simulink model "tesina"  (R2024b)
settings: Solver=VariableStepAuto  StartTime=0.0  StopTime=3  RelTol=1e-3
undefined symbols (not defined in the file or in its folder): ci_core, ci_energia, ci_omp, ci_T_core, ci_T_omp, ci_T_tar, ci_tar, ion, k0, Lz_valuesAzoto, P_tot
libraries: slpidlib x3, simulink x1
settings Model: Creator=feder  LastModifiedBy=costa

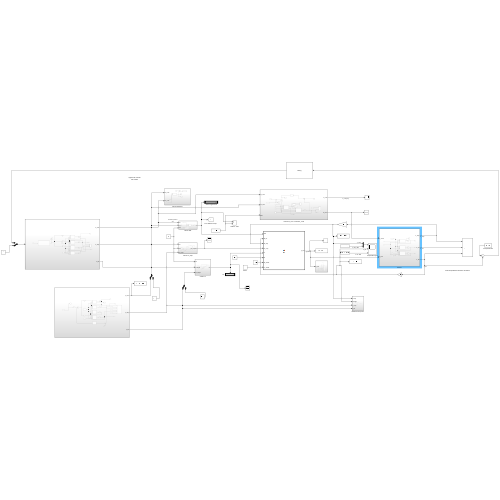
[thumbnail: Simulink's stored preview of the top-level diagram]
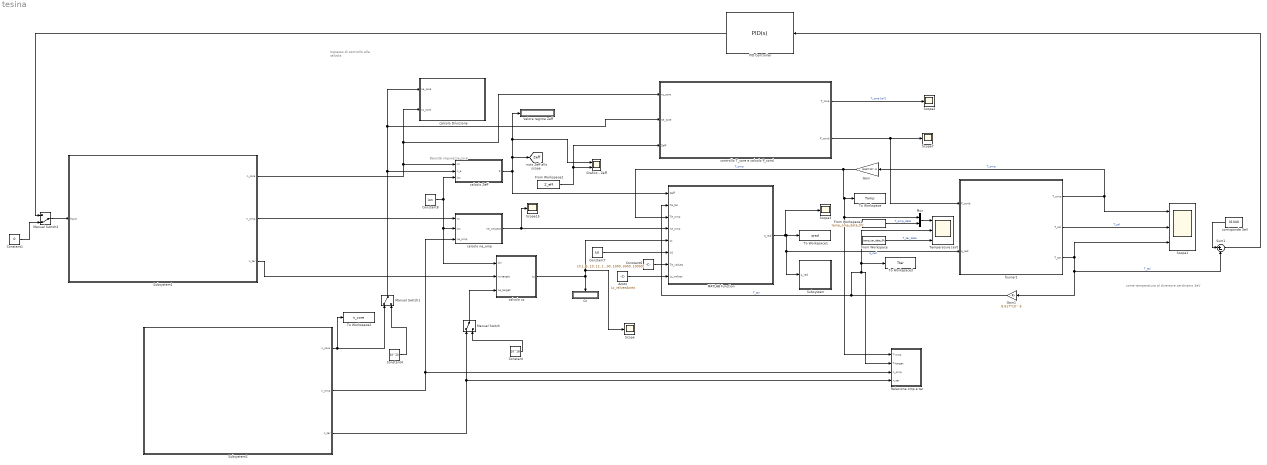
== system tesina ==
  note: come temperatura al divertore cerchiamo 3eV
  note: Ingresso di controllo
      | alla valvola
  note: Densità impurezze
      | core
  Azoto : Constant  Value=Lz_valuesAzoto
  Constant : Constant  Value=10^18
  Constant1 : Constant  Value=0
  Constant4 : Constant  Value=10^20
  Constant6 : Constant  Value=[0,1, 5, 10, 12, 15, 20, 30, 59, 100, 155, 200, 300, 500, 700, 1000, 3000, 10000]
  Constant7 : Constant  Value=k0
  Constant8 : Constant  Value=ion
  Cz : Display
  From Workspace : FromWorkspace  VariableName=temp_tar_data_filt
  From Workspace1 : FromWorkspace  VariableName=temp_omp_data_filt
  From Workspace2 : FromWorkspace  VariableName=Z_eff
  Gain : Gain  Gain=8.617*10^-5
  Gain1 : Gain  Gain=8.617*10^-5
  Grafico - Zeff : Scope  NumInputPorts=2
  MATLAB Function : MATLAB Function  TreatAsAtomicUnit=on
  Manual Switch : ManualSwitch
  Manual Switch1 : ManualSwitch
  Manual Switch2 : ManualSwitch  CurrentSetting=0
  Mux : Mux  Inputs=2
  PID Controller : slpidlib/PID Controller  Controller=PID  Form=Parallel  TimeDomain=Continuous-time  UseExternalTs=off  SampleTime=-1  IntegratorMethod=Forward Euler  FilterMethod=Forward Euler  ControllerParametersSource=internal  P=-5*10^10  I=-0.5*10^8  UseKiTs=off  D=-10^11  UseExternalDerivativeSource=off  N=100  UseFilter=on  TunerSelectOption=Transfer Function Based (PID Tuner App)  InitialConditionSource=internal  InitialConditionForIntegrator=0  InitialConditionForFilter=0  DifferentiatorICPrevScaledInput=0  ExternalReset=none  TrackingMode=off  Kt=1  LimitOutput=off  SatLimitsSource=internal  UpperSaturationLimit=inf  LowerSaturationLimit=-inf  LinearizeAsGain=on  AntiWindupMode=none  Kb=1  LimitIntegrator=off  UpperIntegratorSaturationLimit=inf  LowerIntegratorSaturationLimit=-inf  POutMin=[]  POutMax=[]  IOutMin=[]  IOutMax=[]  DOutMin=[]  DOutMax=[]  NOutMin=[]  NOutMax=[]  SumOutMin=[]  SumOutMax=[]  SaturationOutMin=[]  SaturationOutMax=[]  PParamMin=[]  PParamMax=[]  IParamMin=[]  IParamMax=[]  DParamMin=[]  DParamMax=[]  NParamMin=[]  NParamMax=[]  KbParamMin=[]  KbParamMax=[]  KtParamMin=[]  KtParamMax=[]  KbOutMin=[]  KbOutMax=[]  KtOutMin=[]  KtOutMax=[]  IntegratorOutMin=[]  IntegratorOutMax=[]  FilterOutMin=[]  FilterOutMax=[]  SumI1OutMin=[]  SumI1OutMax=[]  SumI2OutMin=[]  SumI2OutMax=[]  SumI3OutMin=[]  SumI3OutMax=[]  SumI4OutMin=[]  SumI4OutMax=[]  SumDOutMin=[]  SumDOutMax=[]  DifferentiatorOutMin=[]  DifferentiatorOutMax=[]  FilterDiffOutCoefMin=[]  FilterDiffOutCoefMax=[]  ReciprocalOutMin=[]  ReciprocalOutMax=[]  SumDenOutMin=[]  SumDenOutMax=[]  SumNumOutMin=[]  SumNumOutMax=[]  DivideOutMin=[]  DivideOutMax=[]  UdiffTsProdOutMin=[]  UdiffTsProdOutMax=[]  NTsProdOutMin=[]  NTsProdOutMax=[]  UintegralTsProdOutMin=[]  UintegralTsProdOutMax=[]  UngainTsProdOutMin=[]  UngainTsProdOutMax=[]  ClampingZeroOutDataTypeStr=Inherit: Inherit via back propagation  ClampingZeroOutMin=[]  ClampingZeroOutMax=[]  FilterDenConstantOutDataTypeStr=Inherit: Inherit via back propagation  FilterDenConstantOutMin=[]  FilterDenConstantOutMax=[]  PCopyOutDataTypeStr=Inherit: Inherit via back propagation  PCopyOutMin=[]  PCopyOutMax=[]  NCopyOutDataTypeStr=Inherit: Inherit via back propagation  NCopyOutMin=[]  NCopyOutMax=[]  IntegratorContinuousStateAttributes=''  IntegratorStateMustResolveToSignalObject=off  IntegratorRTWStateStorageClass=Auto  FilterContinuousStateAttributes=''  FilterStateMustResolveToSignalObject=off  FilterRTWStateStorageClass=Auto  ParallelPVariant=InternalParameters  IdealPVariant=Disabled  IVariant=InternalParameters  DVariant=InternalParameters  IntegratorVariant=Continuous  SatVariant=Disabled  AWVariant=Passthrough  PCopyVariant=Disabled  TRVariant=Disabled  FdbkBlocksVariant=Forward  IdealPFdbkVariant=Disabled  SatFdbkVariant=Disabled  DerivativeFilterVariant=ContFilter  NVariant=InternalParameters  NCopyVariant=Disabled  FilterICVariant=InternalICsFilter  IntegratorICVariant=InternalICs  ExternalResetVariant=Disabled  TRSumVariant=Passthrough  SumFdbkVariant=Disabled  SumVariant=Sum_PID  TsampFilterVariant=InternalTs  TsampNgainVariant=Passthrough  TsampIntegralVariant=Disabled_SignalSpec  ExternalSaturationOutDataTypeStr=Inherit: Same as second input  DerivativeSourceVariant=ErrorSignal  PreIntVariant=InternalPreInt
  Relazione omp e tar : Subsystem
  Scope{,2..3,7,15} (5 alike) : Scope
  Scope1 : Scope  NumInputPorts=3
  Subsystem : Subsystem
  Subsystem1 : Subsystem
  Subsystem2 : Subsystem
  Sum1 : Sum  Inputs=|+-
  Temperature [eV] : Scope  NumInputPorts=3
  To Workspace : ToWorkspace  VariableName=Tomp  SaveFormat=Timeseries  SampleTime=-1
  To Workspace1 : ToWorkspace  VariableName=qrad  SaveFormat=Timeseries  SampleTime=-1
  To Workspace2 : ToWorkspace  VariableName=n_core  SaveFormat=Timeseries  SampleTime=-1
  To Workspace3 : ToWorkspace  VariableName=Ttar  SaveFormat=Timeseries  SampleTime=-1
  Valore regime Zeff : Display
  calcolo Diluizione : Subsystem
  calcolo Zeff : Subsystem
  calcolo cz : Subsystem
  calcolo ne_omp : Subsystem
  controllo T_core e calcolo P_cond : Subsystem
  corrisponde 3eV : Constant  Value=31340
  fourier1 : Subsystem
  tag scope: Zeff=global
  wires:
  Gain/1 -> MATLAB Function/3(Te_omp), Mux/1, Relazione omp e tar/1(T-omp), To Workspace/1  "T_omp"
  PID Controller/1 -> Manual Switch2/1
  From Workspace1/1 -> Mux/2  "T_omp_data"
  Subsystem2/2(n_omp) -> calcolo ne_omp/3(ne_omp), Relazione omp e tar/3(n_omp)
  Subsystem1/2(n_omp) -> calcolo ne_omp/1(nz)
  Gain1/1 -> Relazione omp e tar/2(T-target), Temperature [eV]/2, To Workspace3/1, MATLAB Function/2(Te_tar)  "T_tar"
  Azoto/1 -> MATLAB Function/8(Lz_values)
  controllo T_core e calcolo P_cond/2(P_cond) -> fourier1/1(P_cond), Scope7/1
  Manual Switch2/1 -> Subsystem1/1(Input)
  Manual Switch/1 -> calcolo cz/3(ne_target)
  Subsystem1/3(n_tar) -> calcolo cz/2(nz-target)
  Subsystem2/3(n_tar) -> Manual Switch/1, Relazione omp e tar/4(n_tar)
  From Workspace2/1 -> controllo T_core e calcolo P_cond/3(Zeff), Grafico - Zeff/2
  Manual Switch1/1 -> controllo T_core e calcolo P_cond/2(ne_core), calcolo Diluizione/1(ne_core), calcolo Zeff/2(n_e)
  Subsystem2/1(n_core) -> Manual Switch1/1, To Workspace2/1
  controllo T_core e calcolo P_cond/1(T_core) -> Scope2/1  "T_core [eV]"
  Constant1/1 -> Manual Switch2/2
  Mux/1 -> Temperature [eV]/1
  Subsystem1/1(n_core) -> calcolo Zeff/1(nz), calcolo Diluizione/2(nz_core), controllo T_core e calcolo P_cond/1(nz_core)
  Constant8/1 -> calcolo cz/1(ion), calcolo ne_omp/2(ion), calcolo Zeff/3(ion)
  From Workspace/1 -> Temperature [eV]/3  "T_tar_data"
  calcolo cz/1(cz) -> Cz/1, Scope/1, MATLAB Function/5(cz)
  MATLAB Function/1(q_rad) -> To Workspace1/1, fourier1/2(q_rad), Subsystem/1(q_rad), Scope3/1  "q_rad"
  corrisponde 3eV/1 -> Sum1/1
  Constant6/1 -> MATLAB Function/7(Te_values)
  Constant/1 -> Manual Switch/2
  Sum1/1 -> PID Controller/1
  calcolo Zeff/1(Z) -> MATLAB Function/1(Zeff), [Zeff], Valore regime Zeff/1, Grafico - Zeff/1
  calcolo ne_omp/1(ne_omptot) -> MATLAB Function/4(ne_omp), Scope15/1
  Constant4/1 -> Manual Switch1/2
  fourier1/3(T_tar) -> Scope1/3, Gain1/1, Sum1/2  "T_tar"
  fourier1/1(T_omp) -> Scope1/1, Gain/1  "T_omp"
  Constant7/1 -> MATLAB Function/6(k0)
  fourier1/2(T_sol) -> Scope1/2  "T_sol"

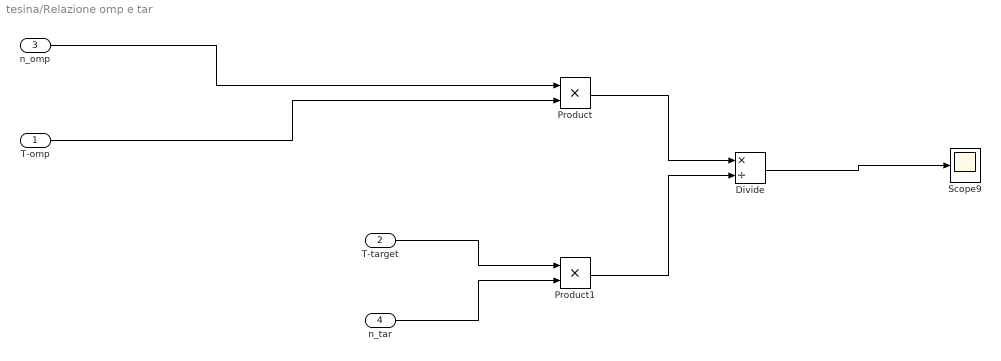
== system tesina/Relazione omp e tar ==
  T-omp : Inport
  T-target : Inport  Port=2
  n_omp : Inport  Port=3
  n_tar : Inport  Port=4
  Divide : Product  Inputs=*/
  Product : Product
  Product1 : Product
  Scope9 : Scope
  wires:
  Product/1 -> Divide/1
  n_tar/1 -> Product1/2
  Divide/1 -> Scope9/1
  Product1/1 -> Divide/2
  n_omp/1 -> Product/1
  T-target/1 -> Product1/1
  T-omp/1 -> Product/2

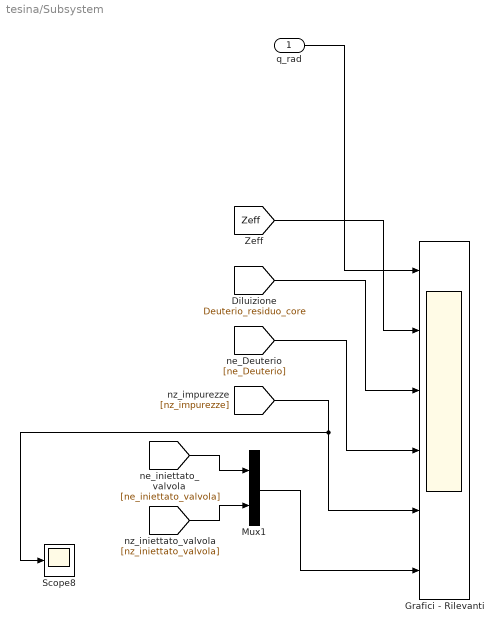
== system tesina/Subsystem ==
  q_rad : Inport
  Grafici - Rilevanti : Scope  NumInputPorts=6
  Mux1 : Mux  Inputs=2
  Scope8 : Scope
  wires:
  q_rad/1 -> Grafici - Rilevanti/1
  [Zeff] -> Grafici - Rilevanti/2
  [nz_impurezze] -> Scope8/1, Grafici - Rilevanti/5
  Mux1/1 -> Grafici - Rilevanti/6
  [nz_iniettato_valvola] -> Mux1/2
  [Deuterio_residuo_core] -> Grafici - Rilevanti/3
  [ne_Deuterio] -> Grafici - Rilevanti/4
  [ne_iniettato_valvola] -> Mux1/1

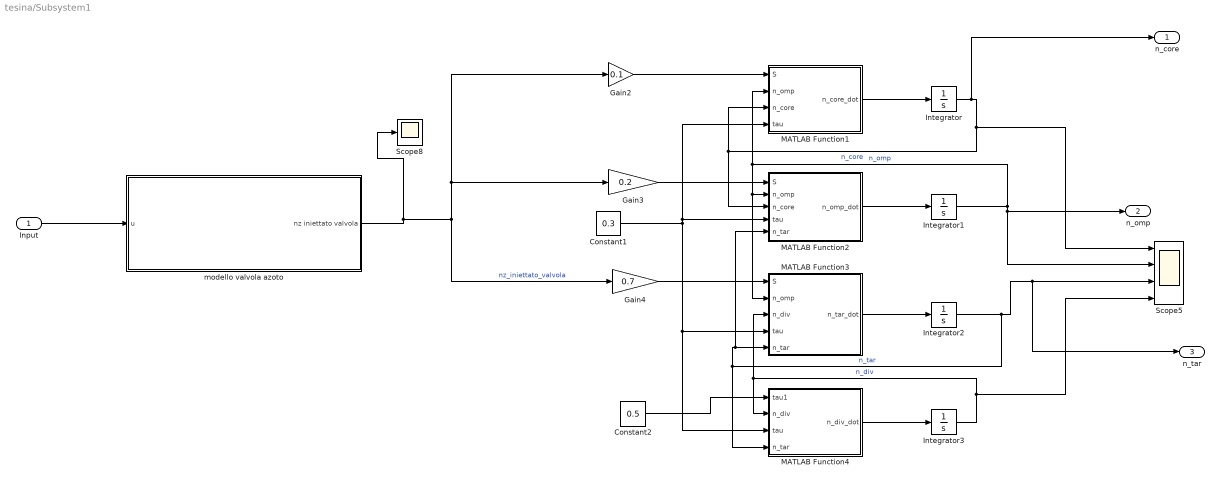
== system tesina/Subsystem1 ==
  Input : Inport
  Constant1 : Constant  Value=0.3
  Constant2 : Constant  Value=0.5
  Gain2 : Gain  Gain=0.1
  Gain3 : Gain  Gain=0.2
  Gain4 : Gain  Gain=0.7
  Integrator{,1..3} (4 alike) : Integrator
  MATLAB Function1 : MATLAB Function  TreatAsAtomicUnit=on
  MATLAB Function2 : MATLAB Function  TreatAsAtomicUnit=on
  MATLAB Function3 : MATLAB Function  TreatAsAtomicUnit=on
  MATLAB Function4 : MATLAB Function  TreatAsAtomicUnit=on
  Scope5 : Scope  NumInputPorts=4
  Scope8 : Scope
  modello valvola azoto : Subsystem
  n_core : Outport
  n_omp : Outport  Port=2
  n_tar : Outport  Port=3
  wires:
  Gain3/1 -> MATLAB Function2/1(S)
  Integrator2/1 -> MATLAB Function4/4(n_tar), MATLAB Function2/5(n_tar), MATLAB Function3/5(n_tar), n_tar/1, Scope5/3  "n_tar"
  MATLAB Function2/1(n_omp_dot) -> Integrator1/1
  Integrator/1 -> n_core/1, Scope5/1, MATLAB Function1/3(n_core), MATLAB Function2/3(n_core)  "n_core"
  Integrator1/1 -> Scope5/2, n_omp/1, MATLAB Function3/2(n_omp), MATLAB Function2/2(n_omp), MATLAB Function1/2(n_omp)  "n_omp"
  Constant1/1 -> MATLAB Function1/4(tau), MATLAB Function2/4(tau), MATLAB Function4/3(tau), MATLAB Function3/4(tau)
  Gain4/1 -> MATLAB Function3/1(S)
  Gain2/1 -> MATLAB Function1/1(S)
  MATLAB Function1/1(n_core_dot) -> Integrator/1
  Integrator3/1 -> Scope5/4, MATLAB Function4/2(n_div), MATLAB Function3/3(n_div)  "n_div"
  MATLAB Function4/1(n_div_dot) -> Integrator3/1
  MATLAB Function3/1(n_tar_dot) -> Integrator2/1
  Constant2/1 -> MATLAB Function4/1(tau1)
  Input/1 -> modello valvola azoto/1(u)
  modello valvola azoto/1(nz iniettato valvola) -> Scope8/1, Gain4/1, Gain3/1, Gain2/1  "nz_iniettato_valvola"

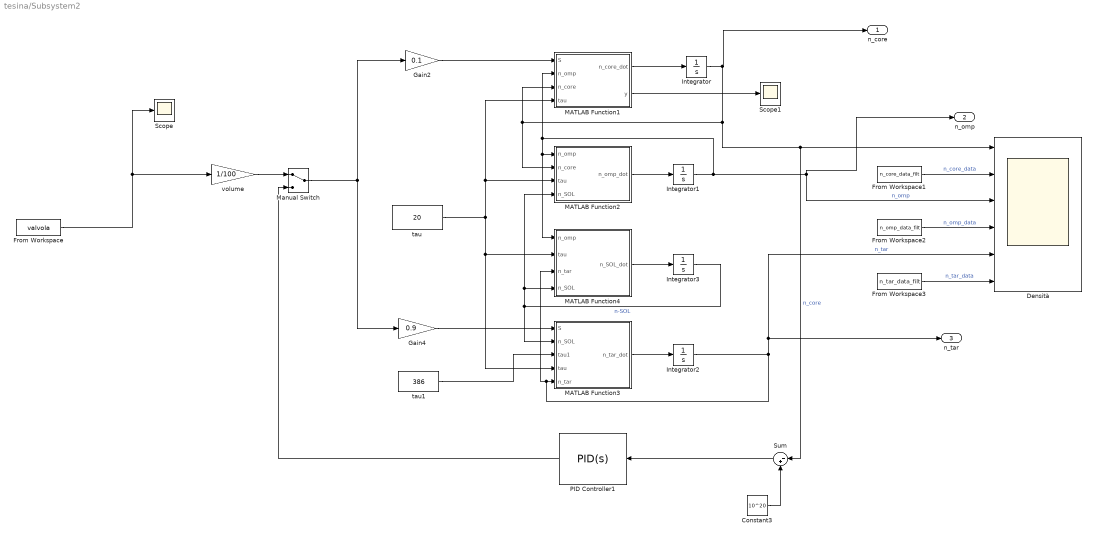
== system tesina/Subsystem2 ==
  Constant3 : Constant  Value=10^20
  Densità : Scope  NumInputPorts=6
  From Workspace : FromWorkspace  VariableName=valvola
  From Workspace1 : FromWorkspace  VariableName=n_core_data_filt
  From Workspace2 : FromWorkspace  VariableName=n_omp_data_filt
  From Workspace3 : FromWorkspace  VariableName=n_tar_data_filt
  Gain2 : Gain  Gain=0.1
  Gain4 : Gain  Gain=0.9
  Integrator : Integrator  InitialCondition=ci_core
  Integrator1 : Integrator  InitialCondition=ci_omp
  Integrator2 : Integrator  InitialCondition=ci_tar
  Integrator3 : Integrator  InitialCondition=(ci_core + ci_tar)/2
  MATLAB Function1 : MATLAB Function  TreatAsAtomicUnit=on
  MATLAB Function2 : MATLAB Function  TreatAsAtomicUnit=on
  MATLAB Function3 : MATLAB Function  TreatAsAtomicUnit=on
  MATLAB Function4 : MATLAB Function  TreatAsAtomicUnit=on
  Manual Switch : ManualSwitch
  PID Controller1 : slpidlib/PID Controller  Controller=PID  Form=Parallel  TimeDomain=Continuous-time  UseExternalTs=off  SampleTime=-1  IntegratorMethod=Forward Euler  FilterMethod=Forward Euler  ControllerParametersSource=internal  P=200  I=606  UseKiTs=off  D=0  UseExternalDerivativeSource=off  N=100  UseFilter=on  TunerSelectOption=Transfer Function Based (PID Tuner App)  InitialConditionSource=internal  InitialConditionForIntegrator=0  InitialConditionForFilter=0  DifferentiatorICPrevScaledInput=0  ExternalReset=none  TrackingMode=off  Kt=1  LimitOutput=off  SatLimitsSource=internal  UpperSaturationLimit=inf  LowerSaturationLimit=-inf  LinearizeAsGain=on  AntiWindupMode=none  Kb=1  LimitIntegrator=off  UpperIntegratorSaturationLimit=inf  LowerIntegratorSaturationLimit=-inf  POutMin=[]  POutMax=[]  IOutMin=[]  IOutMax=[]  DOutMin=[]  DOutMax=[]  NOutMin=[]  NOutMax=[]  SumOutMin=[]  SumOutMax=[]  SaturationOutMin=[]  SaturationOutMax=[]  PParamMin=[]  PParamMax=[]  IParamMin=[]  IParamMax=[]  DParamMin=[]  DParamMax=[]  NParamMin=[]  NParamMax=[]  KbParamMin=[]  KbParamMax=[]  KtParamMin=[]  KtParamMax=[]  KbOutMin=[]  KbOutMax=[]  KtOutMin=[]  KtOutMax=[]  IntegratorOutMin=[]  IntegratorOutMax=[]  FilterOutMin=[]  FilterOutMax=[]  SumI1OutMin=[]  SumI1OutMax=[]  SumI2OutMin=[]  SumI2OutMax=[]  SumI3OutMin=[]  SumI3OutMax=[]  SumI4OutMin=[]  SumI4OutMax=[]  SumDOutMin=[]  SumDOutMax=[]  DifferentiatorOutMin=[]  DifferentiatorOutMax=[]  FilterDiffOutCoefMin=[]  FilterDiffOutCoefMax=[]  ReciprocalOutMin=[]  ReciprocalOutMax=[]  SumDenOutMin=[]  SumDenOutMax=[]  SumNumOutMin=[]  SumNumOutMax=[]  DivideOutMin=[]  DivideOutMax=[]  UdiffTsProdOutMin=[]  UdiffTsProdOutMax=[]  NTsProdOutMin=[]  NTsProdOutMax=[]  UintegralTsProdOutMin=[]  UintegralTsProdOutMax=[]  UngainTsProdOutMin=[]  UngainTsProdOutMax=[]  ClampingZeroOutDataTypeStr=Inherit: Inherit via back propagation  ClampingZeroOutMin=[]  ClampingZeroOutMax=[]  FilterDenConstantOutDataTypeStr=Inherit: Inherit via back propagation  FilterDenConstantOutMin=[]  FilterDenConstantOutMax=[]  PCopyOutDataTypeStr=Inherit: Inherit via back propagation  PCopyOutMin=[]  PCopyOutMax=[]  NCopyOutDataTypeStr=Inherit: Inherit via back propagation  NCopyOutMin=[]  NCopyOutMax=[]  IntegratorContinuousStateAttributes=''  IntegratorStateMustResolveToSignalObject=off  IntegratorRTWStateStorageClass=Auto  FilterContinuousStateAttributes=''  FilterStateMustResolveToSignalObject=off  FilterRTWStateStorageClass=Auto  ParallelPVariant=InternalParameters  IdealPVariant=Disabled  IVariant=InternalParameters  DVariant=InternalParameters  IntegratorVariant=Continuous  SatVariant=Disabled  AWVariant=Passthrough  PCopyVariant=Disabled  TRVariant=Disabled  FdbkBlocksVariant=Forward  IdealPFdbkVariant=Disabled  SatFdbkVariant=Disabled  DerivativeFilterVariant=ContFilter  NVariant=InternalParameters  NCopyVariant=Disabled  FilterICVariant=InternalICsFilter  IntegratorICVariant=InternalICs  ExternalResetVariant=Disabled  TRSumVariant=Passthrough  SumFdbkVariant=Disabled  SumVariant=Sum_PID  TsampFilterVariant=InternalTs  TsampNgainVariant=Passthrough  TsampIntegralVariant=Disabled_SignalSpec  ExternalSaturationOutDataTypeStr=Inherit: Same as second input  DerivativeSourceVariant=ErrorSignal  PreIntVariant=InternalPreInt
  Scope : Scope
  Scope1 : Scope
  Sum : Sum  Inputs=|-+
  tau : Constant  Value=20
  tau1 : Constant  Value=386
  volume : Gain  Gain=1/100
  n_core : Outport
  n_omp : Outport  Port=2
  n_tar : Outport  Port=3
  wires:
  Integrator2/1 -> Densità/5, n_tar/1, MATLAB Function4/3(n_tar), MATLAB Function3/5(n_tar)  "n_tar"
  MATLAB Function2/1(n_omp_dot) -> Integrator1/1
  Integrator/1 -> n_core/1, Sum/1, Densità/1, MATLAB Function1/3(n_core), MATLAB Function2/2(n_core)  "n_core"
  Integrator1/1 -> MATLAB Function4/1(n_omp), MATLAB Function2/1(n_omp), MATLAB Function1/2(n_omp), n_omp/1, Densità/3  "n_omp"
  tau/1 -> MATLAB Function1/4(tau), MATLAB Function2/3(tau), MATLAB Function4/2(tau), MATLAB Function3/4(tau)
  Gain4/1 -> MATLAB Function3/1(S)
  Gain2/1 -> MATLAB Function1/1(S)
  MATLAB Function1/1(n_core_dot) -> Integrator/1
  MATLAB Function3/1(n_tar_dot) -> Integrator2/1
  From Workspace/1 -> volume/1, Scope/1
  From Workspace1/1 -> Densità/2  "n_core_data"
  From Workspace2/1 -> Densità/4  "n_omp_data"
  From Workspace3/1 -> Densità/6  "n_tar_data"
  MATLAB Function1/2(y) -> Scope1/1
  tau1/1 -> MATLAB Function3/3(tau1)
  MATLAB Function4/1(n_SOL_dot) -> Integrator3/1
  Integrator3/1 -> MATLAB Function3/2(n_SOL), MATLAB Function4/4(n_SOL), MATLAB Function2/4(n_SOL)  "n-SOL"
  volume/1 -> Manual Switch/1
  Manual Switch/1 -> Gain4/1, Gain2/1
  Sum/1 -> PID Controller1/1
  Constant3/1 -> Sum/2
  PID Controller1/1 -> Manual Switch/2

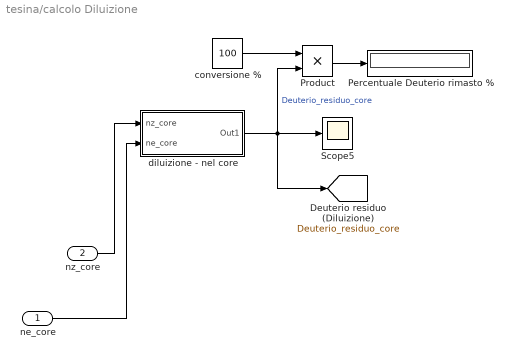
== system tesina/calcolo Diluizione ==
  ne_core : Inport
  nz_core : Inport  Port=2
  Percentuale Deuterio rimasto % : Display
  Product : Product
  Scope5 : Scope
  "conversione % " : Constant  Value=100
  diluizione - nel core : Subsystem
  tag scope: Deuterio_residuo_core=global
  wires:
  Product/1 -> Percentuale Deuterio rimasto %/1
  nz_core/1 -> diluizione - nel core/1(nz_core)
  "conversione % "/1 -> Product/1
  diluizione - nel core/1(Out1) -> [Deuterio_residuo_core], Scope5/1, Product/2  "Deuterio_residuo_core"
  ne_core/1 -> diluizione - nel core/2(ne_core)

== system tesina/calcolo Zeff ==
  note: Tasso di ionizzazione
  note: Desnità impurezze Core
  note: Densità Deuterio Core
  nz : Inport
  n_e : Inport  Port=2
  ion : Inport  Port=3
  MATLAB Function1 : MATLAB Function  TreatAsAtomicUnit=on
  Z : Outport
  wires:
  nz/1 -> MATLAB Function1/1(n_z)
  n_e/1 -> MATLAB Function1/3(n_e)
  ion/1 -> MATLAB Function1/2(ion)
  MATLAB Function1/1(Zeff) -> Z/1

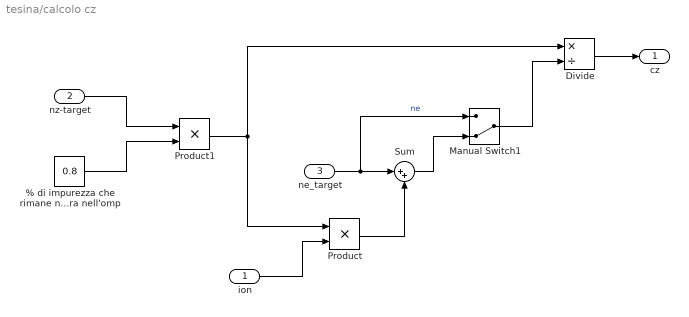
== system tesina/calcolo cz ==
  ion : Inport
  nz-target : Inport  Port=2
  ne_target : Inport  Port=3
  % di impurezza che rimane nel div. Parte restante migra nell'omp : Constant  Value=0.8
  Divide : Product  Inputs=*/
  Manual Switch1 : ManualSwitch  CurrentSetting=0
  Product : Product
  Product1 : Product
  Sum : Sum  Inputs=|++
  cz : Outport
  wires:
  ne_target/1 -> Manual Switch1/1, Sum/1  "ne"
  Sum/1 -> Manual Switch1/2
  Divide/1 -> cz/1
  Manual Switch1/1 -> Divide/2
  Product/1 -> Sum/2
  nz-target/1 -> Product1/1
  % di impurezza che rimane nel div. Parte restante migra nell'omp/1 -> Product1/2
  ion/1 -> Product/2
  Product1/1 -> Divide/1, Product/1

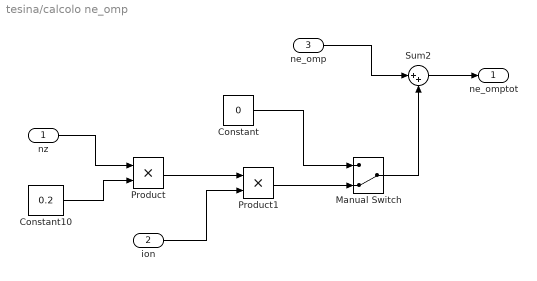
== system tesina/calcolo ne_omp ==
  nz : Inport
  ion : Inport  Port=2
  ne_omp : Inport  Port=3
  Constant : Constant  Value=0
  Constant10 : Constant  Value=0.2
  Manual Switch : ManualSwitch  CurrentSetting=0
  Product : Product
  Product1 : Product
  Sum2 : Sum  Inputs=|++
  ne_omptot : Outport
  wires:
  Constant10/1 -> Product/2
  Sum2/1 -> ne_omptot/1
  nz/1 -> Product/1
  ne_omp/1 -> Sum2/1
  Constant/1 -> Manual Switch/1
  Manual Switch/1 -> Sum2/2
  Product/1 -> Product1/1
  ion/1 -> Product1/2
  Product1/1 -> Manual Switch/2

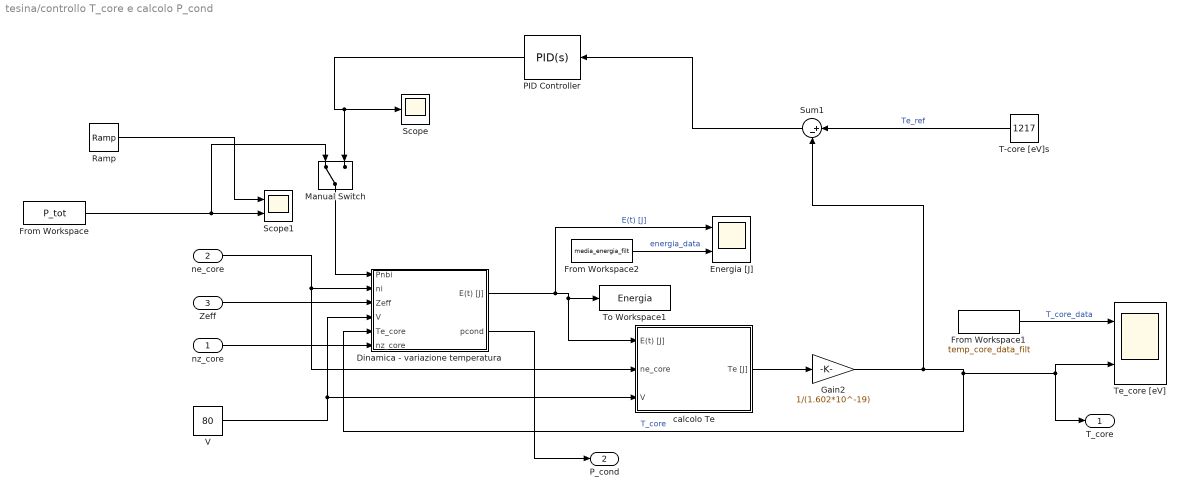
== system tesina/controllo T_core e calcolo P_cond ==
  nz_core : Inport
  ne_core : Inport  Port=2
  Zeff : Inport  Port=3
  Dinamica - variazione temperatura : Subsystem
  Energia [J] : Scope  NumInputPorts=2
  From Workspace : FromWorkspace  VariableName=P_tot
  From Workspace1 : FromWorkspace  VariableName=temp_core_data_filt
  From Workspace2 : FromWorkspace  VariableName=media_energia_filt
  Gain2 : Gain  Gain=1/(1.602*10^-19)
  Manual Switch : ManualSwitch
  PID Controller : slpidlib/PID Controller  Controller=PID  Form=Parallel  TimeDomain=Continuous-time  UseExternalTs=off  SampleTime=-1  IntegratorMethod=Forward Euler  FilterMethod=Forward Euler  ControllerParametersSource=internal  P=100000  I=5000000  UseKiTs=off  D=1  UseExternalDerivativeSource=off  N=3179.8023311838  UseFilter=on  TunerSelectOption=Transfer Function Based (PID Tuner App)  InitialConditionSource=internal  InitialConditionForIntegrator=0  InitialConditionForFilter=0  DifferentiatorICPrevScaledInput=0  ExternalReset=none  TrackingMode=off  Kt=1  LimitOutput=off  SatLimitsSource=internal  UpperSaturationLimit=inf  LowerSaturationLimit=-inf  LinearizeAsGain=on  AntiWindupMode=none  Kb=1  LimitIntegrator=off  UpperIntegratorSaturationLimit=inf  LowerIntegratorSaturationLimit=-inf  POutMin=[]  POutMax=[]  IOutMin=[]  IOutMax=[]  DOutMin=[]  DOutMax=[]  NOutMin=[]  NOutMax=[]  SumOutMin=[]  SumOutMax=[]  SaturationOutMin=[]  SaturationOutMax=[]  PParamMin=[]  PParamMax=[]  IParamMin=[]  IParamMax=[]  DParamMin=[]  DParamMax=[]  NParamMin=[]  NParamMax=[]  KbParamMin=[]  KbParamMax=[]  KtParamMin=[]  KtParamMax=[]  KbOutMin=[]  KbOutMax=[]  KtOutMin=[]  KtOutMax=[]  IntegratorOutMin=[]  IntegratorOutMax=[]  FilterOutMin=[]  FilterOutMax=[]  SumI1OutMin=[]  SumI1OutMax=[]  SumI2OutMin=[]  SumI2OutMax=[]  SumI3OutMin=[]  SumI3OutMax=[]  SumI4OutMin=[]  SumI4OutMax=[]  SumDOutMin=[]  SumDOutMax=[]  DifferentiatorOutMin=[]  DifferentiatorOutMax=[]  FilterDiffOutCoefMin=[]  FilterDiffOutCoefMax=[]  ReciprocalOutMin=[]  ReciprocalOutMax=[]  SumDenOutMin=[]  SumDenOutMax=[]  SumNumOutMin=[]  SumNumOutMax=[]  DivideOutMin=[]  DivideOutMax=[]  UdiffTsProdOutMin=[]  UdiffTsProdOutMax=[]  NTsProdOutMin=[]  NTsProdOutMax=[]  UintegralTsProdOutMin=[]  UintegralTsProdOutMax=[]  UngainTsProdOutMin=[]  UngainTsProdOutMax=[]  ClampingZeroOutDataTypeStr=Inherit: Inherit via back propagation  ClampingZeroOutMin=[]  ClampingZeroOutMax=[]  FilterDenConstantOutDataTypeStr=Inherit: Inherit via back propagation  FilterDenConstantOutMin=[]  FilterDenConstantOutMax=[]  PCopyOutDataTypeStr=Inherit: Inherit via back propagation  PCopyOutMin=[]  PCopyOutMax=[]  NCopyOutDataTypeStr=Inherit: Inherit via back propagation  NCopyOutMin=[]  NCopyOutMax=[]  IntegratorContinuousStateAttributes=''  IntegratorStateMustResolveToSignalObject=off  IntegratorRTWStateStorageClass=Auto  FilterContinuousStateAttributes=''  FilterStateMustResolveToSignalObject=off  FilterRTWStateStorageClass=Auto  ParallelPVariant=InternalParameters  IdealPVariant=Disabled  IVariant=InternalParameters  DVariant=InternalParameters  IntegratorVariant=Continuous  SatVariant=Disabled  AWVariant=Passthrough  PCopyVariant=Disabled  TRVariant=Disabled  FdbkBlocksVariant=Forward  IdealPFdbkVariant=Disabled  SatFdbkVariant=Disabled  DerivativeFilterVariant=ContFilter  NVariant=InternalParameters  NCopyVariant=Disabled  FilterICVariant=InternalICsFilter  IntegratorICVariant=InternalICs  ExternalResetVariant=Disabled  TRSumVariant=Passthrough  SumFdbkVariant=Disabled  SumVariant=Sum_PID  TsampFilterVariant=InternalTs  TsampNgainVariant=Passthrough  TsampIntegralVariant=Disabled_SignalSpec  ExternalSaturationOutDataTypeStr=Inherit: Same as second input  DerivativeSourceVariant=ErrorSignal  PreIntVariant=InternalPreInt
  Ramp : simulink/Sources/Ramp  slope=380436  start=0  InitialOutput=P_tot.Data(1)
  Scope : Scope
  Scope1 : Scope  NumInputPorts=2
  Sum1 : Sum  Inputs=|+-
  T-core [eV]s : Constant  Value=1217
  Te_core [eV] : Scope  NumInputPorts=2
  To Workspace1 : ToWorkspace  VariableName=Energia  SaveFormat=Timeseries  SampleTime=-1
  V : Constant  Value=80
  calcolo Te : Subsystem
  T_core : Outport
  P_cond : Outport  Port=2
  wires:
  T-core [eV]s/1 -> Sum1/1  "Te_ref"
  Gain2/1 -> Sum1/2, Dinamica - variazione temperatura/5(Te_core), T_core/1, Te_core [eV]/2  "T_core"
  Zeff/1 -> Dinamica - variazione temperatura/3(Zeff)
  ne_core/1 -> calcolo Te/2(ne_core), Dinamica - variazione temperatura/2(ni)
  V/1 -> calcolo Te/3(V), Dinamica - variazione temperatura/4(V)
  Dinamica - variazione temperatura/1(E(t) [J]) -> Energia [J]/1, calcolo Te/1(E(t) [J]), To Workspace1/1  "E(t) [J]"
  Sum1/1 -> PID Controller/1
  PID Controller/1 -> Manual Switch/2, Scope/1
  nz_core/1 -> Dinamica - variazione temperatura/6(nz_core)
  Dinamica - variazione temperatura/2(pcond) -> P_cond/1
  calcolo Te/1(Te [J]) -> Gain2/1
  Ramp/1 -> Scope1/1
  Manual Switch/1 -> Dinamica - variazione temperatura/1(Pnbi)
  From Workspace/1 -> Manual Switch/1, Scope1/2
  From Workspace1/1 -> Te_core [eV]/1  "T_core_data"
  From Workspace2/1 -> Energia [J]/2  "energia_data"

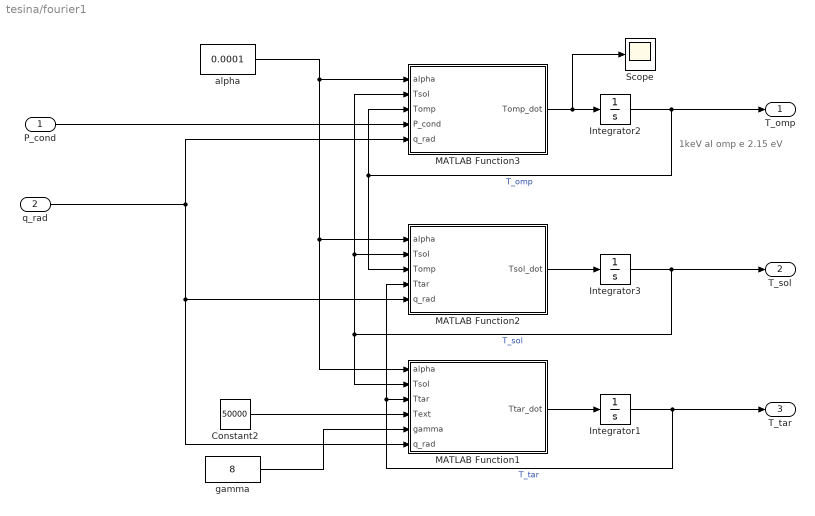
== system tesina/fourier1 ==
  note: 1keV al omp e 2.15 eV
  P_cond : Inport
  q_rad : Inport  Port=2
  Constant2 : Constant  Value=50000
  Integrator1 : Integrator  InitialCondition=ci_T_tar/(8.617*10^-5)
  Integrator2 : Integrator  InitialCondition=ci_T_omp/(8.617*10^-5)
  Integrator3 : Integrator  InitialCondition=(ci_T_core + ci_T_omp)/( 2*8.617*10^-5)
  MATLAB Function1 : MATLAB Function  TreatAsAtomicUnit=on
  MATLAB Function2 : MATLAB Function  TreatAsAtomicUnit=on
  MATLAB Function3 : MATLAB Function  TreatAsAtomicUnit=on
  Scope : Scope
  alpha : Constant  Value=0.0001
  gamma : Constant  Value=8  VectorParams1D=off
  T_omp : Outport
  T_sol : Outport  Port=2
  T_tar : Outport  Port=3
  wires:
  alpha/1 -> MATLAB Function1/1(alpha), MATLAB Function2/1(alpha), MATLAB Function3/1(alpha)
  MATLAB Function3/1(Tomp_dot) -> Scope/1, Integrator2/1
  Constant2/1 -> MATLAB Function1/4(Text)
  Integrator1/1 -> T_tar/1, MATLAB Function2/4(Ttar), MATLAB Function1/3(Ttar)  "T_tar"
  P_cond/1 -> MATLAB Function3/4(P_cond)
  q_rad/1 -> MATLAB Function3/5(q_rad), MATLAB Function2/5(q_rad), MATLAB Function1/6(q_rad)
  gamma/1 -> MATLAB Function1/5(gamma)
  MATLAB Function2/1(Tsol_dot) -> Integrator3/1
  MATLAB Function1/1(Ttar_dot) -> Integrator1/1
  Integrator2/1 -> T_omp/1, MATLAB Function3/3(Tomp), MATLAB Function2/3(Tomp)  "T_omp"
  Integrator3/1 -> MATLAB Function3/2(Tsol), MATLAB Function2/2(Tsol), MATLAB Function1/2(Tsol), T_sol/1  "T_sol"

== system tesina/Subsystem1/modello valvola azoto ==
  u : Inport
  Saturation : Saturate  UpperLimit=inf  LowerLimit=0
  Transfer Fcn : TransferFcn  Numerator=[0.91]  Denominator=[0.002 1]
  Transport Delay : TransportDelay  DelayTime=0.0019
  nz iniettato valvola : Outport
  wires:
  Transfer Fcn/1 -> Saturation/1  "nz"
  Transport Delay/1 -> Transfer Fcn/1
  u/1 -> Transport Delay/1
  Saturation/1 -> nz iniettato valvola/1

== system tesina/calcolo Diluizione/diluizione - nel core ==
  nz_core : Inport
  ne_core : Inport  Port=2
  Divide : Product  Inputs=/*
  Product : Product
  Subtract : Sum  Inputs=+-
  Tasso di ionizzazione : Constant  Value=ion
  Out1 : Outport
  wires:
  nz_core/1 -> Product/1
  Tasso di ionizzazione/1 -> Product/2
  ne_core/1 -> Subtract/1, Divide/1
  Product/1 -> Subtract/2
  Divide/1 -> Out1/1
  Subtract/1 -> Divide/2

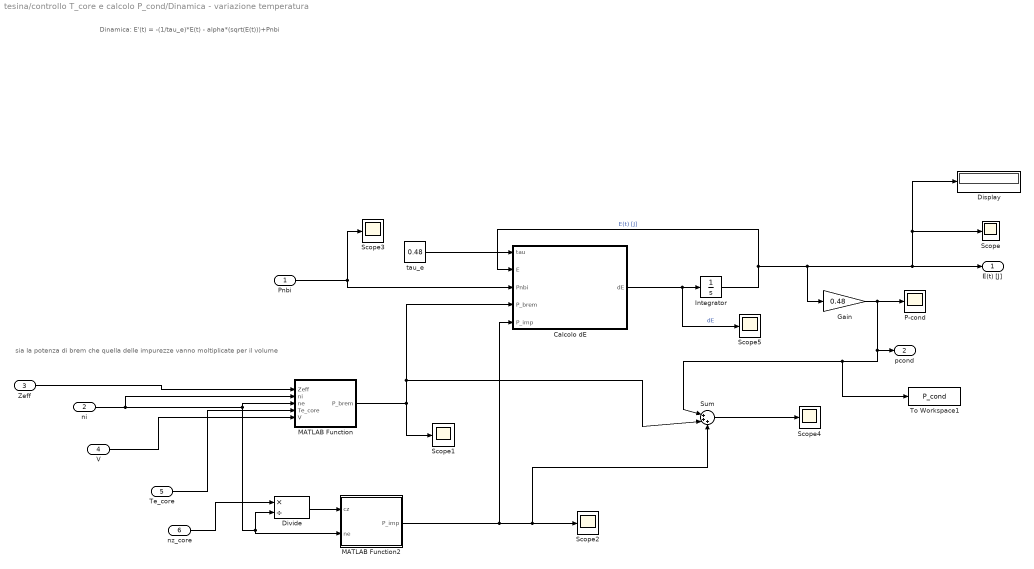
== system tesina/controllo T_core e calcolo P_cond/Dinamica - variazione temperatura ==
  note: sia la potenza di brem che quella delle impurezze vanno moltiplicate per il volume
  note: Dinamica: E'(t) = -(1/tau_e)*E(t) - alpha*(sqrt(E(t)))+Pnbi
  Pnbi : Inport
  ni : Inport  Port=2
  Zeff : Inport  Port=3
  V : Inport  Port=4
  Te_core : Inport  Port=5
  nz_core : Inport  Port=6
  Calcolo dE : MATLAB Function  TreatAsAtomicUnit=on
  Display : Display
  Divide : Product  Inputs=*/
  Gain : Gain  Gain=0.48
  Integrator : Integrator  InitialCondition=ci_energia
  MATLAB Function : MATLAB Function  TreatAsAtomicUnit=on
  MATLAB Function2 : MATLAB Function  TreatAsAtomicUnit=on
  P-cond : Scope
  Scope{,1..5} (6 alike) : Scope
  Sum : Sum  Inputs=|+++
  To Workspace1 : ToWorkspace  VariableName=P_cond  SaveFormat=Timeseries  SampleTime=-1
  tau_e : Constant  Value=0.48
  E(t) [J] : Outport
  pcond : Outport  Port=2
  wires:
  Calcolo dE/1(dE) -> Scope5/1, Integrator/1  "dE"
  tau_e/1 -> Calcolo dE/1(tau)
  ni/1 -> MATLAB Function/2(ni), MATLAB Function2/2(ne), Divide/2, MATLAB Function/3(ne)
  Zeff/1 -> MATLAB Function/1(Zeff)
  Pnbi/1 -> Scope3/1, Calcolo dE/3(Pnbi)
  Integrator/1 -> Calcolo dE/2(E), Gain/1, Display/1, Scope/1, E(t) [J]/1  "E(t) [J]"
  MATLAB Function/1(P_brem) -> Calcolo dE/4(P_brem), Sum/2, Scope1/1
  Te_core/1 -> MATLAB Function/4(Te_core)
  nz_core/1 -> Divide/1
  Divide/1 -> MATLAB Function2/1(cz)
  MATLAB Function2/1(P_imp) -> Calcolo dE/5(P_imp), Sum/3, Scope2/1
  Gain/1 -> To Workspace1/1, Sum/1, pcond/1, P-cond/1
  Sum/1 -> Scope4/1
  V/1 -> MATLAB Function/5(V)

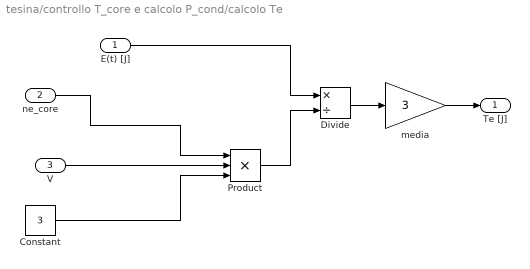
== system tesina/controllo T_core e calcolo P_cond/calcolo Te ==
  E(t) [J] : Inport
  ne_core : Inport  Port=2
  V : Inport  Port=3
  Constant : Constant  Value=3
  Divide : Product  Inputs=*/
  Product : Product  Inputs=3
  media : Gain  Gain=3
  Te [J] : Outport
  wires:
  V/1 -> Product/2
  Constant/1 -> Product/3
  E(t) [J]/1 -> Divide/1
  Product/1 -> Divide/2
  Divide/1 -> media/1
  ne_core/1 -> Product/1
  media/1 -> Te [J]/1

== matlab function tesina/controllo T_core e calcolo P_cond/Dinamica - variazione temperatura/MATLAB Function ==
  data: Zeff input; P_brem output; ni input; ne input; Te_core input; V input
function P_brem = fcn(Zeff, ni, ne,Te_core,V)
    P_brem = (1.7*10^-38)*Zeff^2*ni*ne*sqrt(Te_core)*V;
end

== matlab function tesina/Subsystem1/MATLAB Function4 ==
  data: tau1 input; n_div_dot output; n_div input; tau input; n_tar input
function n_div_dot = fcn(tau1,n_div,tau, n_tar)
    n_div_dot =  (n_tar-n_div)/20-(n_div)/tau1;
end

== matlab function tesina/fourier1/MATLAB Function1 ==
  data: alpha input; Ttar_dot output; Tsol input; Ttar input; Text input; gamma input; q_rad input
function Ttar_dot = fun(alpha, Tsol, Ttar, Text, gamma,q_rad)
  Ttar_dot = (Tsol-Ttar)*alpha+(Text-Ttar)*gamma-q_rad/9 
end

== matlab function tesina/fourier1/MATLAB Function2 ==
  data: alpha input; Tsol_dot output; Tsol input; Tomp input; Ttar input; q_rad input
function Tsol_dot = fun(alpha, Tsol, Tomp, Ttar,q_rad)
    Tsol_dot = (Tomp-Tsol)*alpha+(Ttar-Tsol)*alpha-q_rad/(3*3)
end

== matlab function tesina/fourier1/MATLAB Function3 ==
  data: alpha input; Tomp_dot output; Tsol input; Tomp input; P_cond input; q_rad input
function Tomp_dot = fun(alpha , Tsol,Tomp,P_cond,q_rad)
    Tomp_dot = (Tsol-Tomp)*alpha+(P_cond)/(1000*0.014*3)-q_rad/(3*3)

end

== matlab function tesina/Subsystem2/MATLAB Function1 ==
  data: S input; n_core_dot output; n_omp input; n_core input; tau input; y output
function [n_core_dot,y] = fcn(S, n_omp,n_core,tau)
    n_core_dot =  S+(n_omp-n_core)/tau;
    y = (n_omp-n_core)/tau
end

== matlab function tesina/Subsystem2/MATLAB Function2 ==
  data: n_omp_dot output; n_omp input; n_core input; tau input; n_SOL input
function n_omp_dot = fcn( n_omp,n_core,tau, n_SOL)
    n_omp_dot =  (n_core-n_omp)/tau+(n_SOL-n_omp)/tau ;
    %n_omp_dot =  S+(n_tar-n_omp)/8 ;
end

== matlab function tesina/calcolo Zeff/MATLAB Function1 ==
  data: n_z input; Zeff output; ion input; n_e input
function Zeff = fcn(n_z,ion, n_e)
  
    %Zeff = 2 + (n_z*ion^2+n_e)/(n_z*ion+n_e);

    Zeff = 0.4 + (n_z*ion^2+n_e)/(n_z*ion+n_e)
    
end

== matlab function tesina/Subsystem2/MATLAB Function3 ==
  data: S input; n_tar_dot output; n_SOL input; tau1 input; tau input; n_tar input
function n_tar_dot = fcn(S, n_SOL,tau1, tau, n_tar)
    n_tar_dot =  S+(n_SOL-n_tar)/tau-n_tar/tau1;
end

== matlab function tesina/MATLAB Function ==
  data: q_rad output; Zeff input; Te_tar input; Te_omp input; ne_omp input; cz input; k0 input; Te_values input; Lz_values input
function q_rad = fcn(Zeff, Te_tar, Te_omp, ne_omp, cz, k0, Te_values, Lz_values)

    % Usa interp1 per fare l'interpolazione
    Lz = @(Te) interp1(Te_values, Lz_values, Te, 'pchip', 'extrap');
    % Definisci l'integranda come una funzione anonima
    integrand = @(Te) Lz(Te) .* Te.^0.5 .* Zeff.^(-0.3);
    %disp(integrand)
    % Calcola l'integrale numerico tra Te_tar e Te_omp
    y = integral(integrand, Te_tar, Te_omp);
    %disp(y)
    %disp(cz)
    q_rad = ne_omp*Te_omp*sqrt(2*max(0,cz*k0*y));
    %disp(q_rad)

end

== matlab function tesina/Subsystem2/MATLAB Function4 ==
  data: n_SOL_dot output; n_omp input; tau input; n_tar input; n_SOL input
function n_SOL_dot = fcn( n_omp, tau, n_tar, n_SOL)
    n_SOL_dot =  (n_omp-n_SOL)/tau+(n_tar-n_SOL)/tau;
end

== matlab function tesina/controllo T_core e calcolo P_cond/Dinamica - variazione temperatura/MATLAB Function2 ==
  data: cz input; ne input; P_imp output
function P_imp = fcn(cz, ne)
    P_imp = cz*ne^2*(10^-34)
end

== matlab function tesina/Subsystem1/MATLAB Function1 ==
  data: S input; n_core_dot output; n_omp input; n_core input; tau input
function n_core_dot = fcn(S, n_omp,n_core,tau)
    n_core_dot =  S+(n_omp-n_core)/8000;
end

== matlab function tesina/Subsystem1/MATLAB Function2 ==
  data: S input; n_omp_dot output; n_omp input; n_core input; tau input; n_tar input
function n_omp_dot = fcn(S, n_omp,n_core,tau, n_tar)
    n_omp_dot =  S+(n_core-n_omp)/800+(n_tar-n_omp)/200 ;
    %n_omp_dot =  S+(n_tar-n_omp)/8 ;
end

== matlab function tesina/Subsystem1/MATLAB Function3 ==
  data: S input; n_tar_dot output; n_omp input; n_div input; tau input; n_tar input
function n_tar_dot = fcn(S, n_omp,n_div,tau, n_tar)
    n_tar_dot =  S+(n_omp-n_tar)/200+(n_div-n_tar)/20;
end

== matlab function tesina/controllo T_core e calcolo P_cond/Dinamica - variazione temperatura/Calcolo dE ==
  data: tau input; E input; dE output; Pnbi input; P_brem input; P_imp input
function dE  = eqDiff(tau, E, Pnbi, P_brem, P_imp)

    % delta = 1e-8; % Se E < soglia, => E = 0
    % k = 10;
    % stopSim = false;
    % 
    % if E < delta
    %     dE = 0;
    %     %stopSim = true; 
    % 
    % else
    dE = -(1/tau)*E + Pnbi -P_brem -P_imp;
    %le impurezze al momento sono nulle 
        
    % end
    % 
end
